simulink model "prob_8"  (R2020b)
settings: Solver=VariableStepAuto  StartTime=0.0  StopTime=10.0  RelTol=1e-3
settings Model: Creator=Lakshmi  LastModifiedBy=Lakshmi

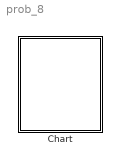
== system prob_8 ==
  Chart : Stateflow chart  TreatAsAtomicUnit=on

== stateflow chart prob_8/Chart ==
  state Idle
    en:m=0;
  state Door_Closed
    en:c=1;
  state Up
    en:m=1;
    during:f=f+1;
  state Down
    en:m=-1;
    during:f=f-1;
  state Stop
    en:m=0;
    c=1;
    during:m=0
  state Door_Open
    en:c=0;
    during:c=0;
    m=0;
  (default) -> Idle
